simulink model "c_piLine_loadVarR"  (R2024b)
settings: Solver=VariableStepAuto  StartTime=0.0  StopTime=Tsim  RelTol=1e-3
libraries: nesl_utility x6, fl_lib x4, ODEsim x2
settings Model: Creator=cao2851  LastModifiedBy=cao2851
settings DataIOCC: ExternalInput=ds{1}  LoadExternalInput=on

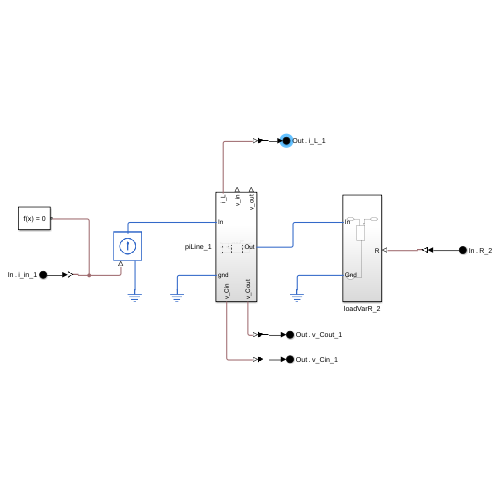
[thumbnail: Simulink's stored preview of the top-level diagram]
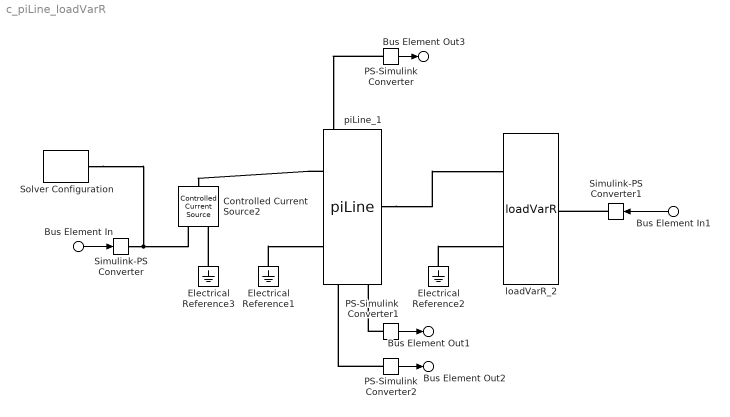
== system c_piLine_loadVarR ==
  Bus Element In : Inport  PortName=In  Element=i_in_1
  Bus Element In1 : Inport  PortName=In  Element=R_2
  Controlled Current Source2 : fl_lib/Electrical/Electrical Sources/Controlled Current Source
  Electrical Reference1 : fl_lib/Electrical/Electrical Elements/Electrical Reference
  Electrical Reference2 : fl_lib/Electrical/Electrical Elements/Electrical Reference
  Electrical Reference3 : fl_lib/Electrical/Electrical Elements/Electrical Reference
  PS-Simulink Converter : nesl_utility/PS-Simulink Converter  PhysicalDomain=network_engine_domain  SubClassName=ps_output  LeftPortType=input  RightPortType=output  PseudoPeriodic=off  Frequencies=[]  VectorFormat=inherit  Unit=inherit  AffineConversion=off
  PS-Simulink Converter1 : nesl_utility/PS-Simulink Converter  PhysicalDomain=network_engine_domain  SubClassName=ps_output  LeftPortType=input  RightPortType=output  PseudoPeriodic=off  Frequencies=[]  VectorFormat=inherit  Unit=inherit  AffineConversion=off
  PS-Simulink Converter2 : nesl_utility/PS-Simulink Converter  PhysicalDomain=network_engine_domain  SubClassName=ps_output  LeftPortType=input  RightPortType=output  PseudoPeriodic=off  Frequencies=[]  VectorFormat=inherit  Unit=inherit  AffineConversion=off
  Simulink-PS Converter : nesl_utility/Simulink-PS Converter  PhysicalDomain=network_engine_domain  SubClassName=ps_input  LeftPortType=input  RightPortType=output  PseudoPeriodic=off  Frequencies=[]  NoiseDistribution=none  NoiseParameters=[]  Unit=1  AffineConversion=off  FilteringAndDerivatives=provide  SimscapeFilterOrder=1  InputFilterTimeConstant=0.001  UdotUserProvided=0
  Simulink-PS Converter1 : nesl_utility/Simulink-PS Converter  PhysicalDomain=network_engine_domain  SubClassName=ps_input  LeftPortType=input  RightPortType=output  PseudoPeriodic=off  Frequencies=[]  NoiseDistribution=none  NoiseParameters=[]  Unit=1  AffineConversion=off  FilteringAndDerivatives=provide  SimscapeFilterOrder=1  InputFilterTimeConstant=0.001  UdotUserProvided=0
  Solver Configuration : nesl_utility/Solver Configuration  PhysicalDomain=network_engine_domain  SubClassName=solver  LeftPortType=input  RightPortType=generic  Tones=[]  Harmonics=[]  SimulateNoise=off  Profile=off  UseLocalSampling=off  EnableSwitchedLinearOptims=on  FrequencyDomain=off  UseCCode=off  RelTol=0.001  AbsTol=0.001  MinStep=1e-09  ToWorkspace=off  RevertToSquareIcSolve=off  NumHomotopyIterations=100  PhasorMode=off  PhasorModeNumHarmonics=1  ConsistencySolver=NEWTON_XTOL_AFTER_FTOL  IndexReductionMethod=DerivativeReplacement  DoDC=off  ResidualTolerance=1e-09  ConsistencyTolSource=GLOBAL  ConsistencyAbsTol=0.001  ConsistencyRelTol=0.001  ConsistencyTolFactor=1e-6  UseLocalSolver=on  LocalSolverChoice=NE_BACKWARD_EULER_ADVANCER  ResolveIndetEquations=on  FunctionEvalNumThread=1  LocalSolverSampleTime=dtMax  DoFixedCost=off  MaxNonlinIter=3  MaxModeIter=2  ComputeImpulses=off  ImpulseIterations=2  LinearAlgebra=auto  LinearAlgebraNumThread=0  EquationFormulation=NE_TIME_EF  DelaysMemoryBudget=1024  AutomaticFiltering=on  FilteringTimeConstant=0.001  PartitionStorageMethod=AS_NEEDED  PartitionMemoryBudget=1024  PartitionMethod=ROBUST  MultibodyUseLocalSolver=off  MultibodyLocalSolverChoice=ODE1  MultibodyLocalSolverSampleTime=0.001
  loadVarR_2 : ODEsim/loadVarR  SystemSampleTime=-1  VariantActivationTime=update diagram  AllowFlexibleInterface=on  Latency=0  AutoFrameSizeCalculation=off
  piLine_1 : ODEsim/piLine  SystemSampleTime=-1  VariantActivationTime=update diagram  AllowFlexibleInterface=on  Latency=0  AutoFrameSizeCalculation=off
      link override Cline1: c=C_1 / 2 * Len_1
      link override Cline1_r: R=R_c_1
      link override Cline2: c=C_1 / 2 * Len_1
      link override Cline2_r: R=R_c_1
      link override Lline: l=L_1 * Len_1
      link override Rline: R=R_1 * Len_1
      settings: PortSchema="{\"entries\":[{\"content\":{\"sides\":[{\"content\":{\"connectorIds\":[\"LConn1\",\"LConn2\"]},\"type\":\"ConnectorPlacement.EquallySpacedRectSide\",\"uuid\":\"2f581a64-5488-4115-8fb4-4c7dc7f7cc02\"},{\"content\":{\"connectorIds\":[\"RConn1\"],\"side\":\"RIGHT\"},\"type\":\"ConnectorPlacement.EquallySpacedRectSide\",\"uuid\":\"41fc3ed1-c08d-4cec-81c4-9e5ea37f4b50\"},{\"content\":{\"connectorIds\":[\"LConn3\",\"LConn4\",\"LConn5\"],\"side\":\"TOP\"},\"type\":\"ConnectorPlacement.EquallySpacedRectSide\",\"uuid\":\"f632da0e-7244-44f2-8232-d25344579225\"},{\"content\":{\"connectorIds\":[\"RConn2\",\"RConn3\"],\"side\":\"BOTTOM\"},\"type\":\"ConnectorPlacement.EquallySpacedRectSide\",\"uuid\":\"4895b748-0fce-4270-baa5-001cc2b4bab4\"}]},\"type\":\"ConnectorPlacement.EquallySpacedConnector\",\"uuid\":\"08f1579d-6e1b-4490-ba48-7710ed18f2cd\"}],\"packageUris\":[\"http://schema.mathworks.com/mf0/Connector/R2020b\"],\"version\":\"1.0\"}"
  Bus Element Out1 : Outport  PortName=Out  Element=v_Cout_1
  Bus Element Out2 : Outport  PortName=Out  Element=v_Cin_1
  Bus Element Out3 : Outport  PortName=Out  Element=i_L_1
  wires:
  Bus Element In/1 -> Simulink-PS Converter/1
  Bus Element In1/1 -> Simulink-PS Converter1/1
  PS-Simulink Converter2/1 -> Bus Element Out2/1
  PS-Simulink Converter1/1 -> Bus Element Out1/1
  PS-Simulink Converter/1 -> Bus Element Out3/1
  connections:
  Simulink-PS Converter/RConn1 -- Controlled Current Source2/RConn1 -- Solver Configuration/RConn1
  piLine_1/LConn1 -- Controlled Current Source2/LConn1
  PS-Simulink Converter1/LConn1 -- piLine_1/RConn3
  PS-Simulink Converter2/LConn1 -- piLine_1/RConn2
  PS-Simulink Converter/LConn1 -- piLine_1/LConn3
  Electrical Reference1/LConn1 -- piLine_1/LConn2
  Electrical Reference3/LConn1 -- Controlled Current Source2/RConn2
  piLine_1/RConn1 -- loadVarR_2/LConn1
  Electrical Reference2/LConn1 -- loadVarR_2/LConn2
  Simulink-PS Converter1/RConn1 -- loadVarR_2/RConn1
